simulink model "LQR_MPC_comparison"  (R2023a)
settings: Solver=VariableStepAuto  StartTime=0.0  StopTime=3  RelTol=1e-3
values from neighbouring files (symbols this model uses):
  B_tilda = [sysdis.B(1) Bw_bar(1,1) Bw_bar(1,2); sysdis.B(2) Bw_bar(2,1) Bw_bar(2,2)]    [motor.m]
  D_tilda = [0 0 0 ; 0 0 0]    [motor.m]
  N = 10    [motor.m]    (also in motor_mpc.m = 3; mpc_unconstrained.m)
  Q_LQ = eye(2)    [motor.m]
  R_LQ = 1    [motor.m]
  sysdis = c2d(sys,Ts)    [motor.m]
  Ts = 0.001    [parameters.m]
  u_max = 12    [constraints.m]
  u_min = 0    [constraints.m]
  uBar = -(A(1,1)*(-A(2,2)*nref/A(2,1)) + A(1,2)*nref)*L    [motor.m]
  w = [1 1]'    [parameters.m]
  x0 = [0.2 70.3]'    [motor.m]
  yref = [iref nref]'    [motor.m]
undefined symbols (not defined in the file or in its folder): Kd, motor_mpc, Sd
settings Model: Creator=Diego  LastModifiedBy=paul

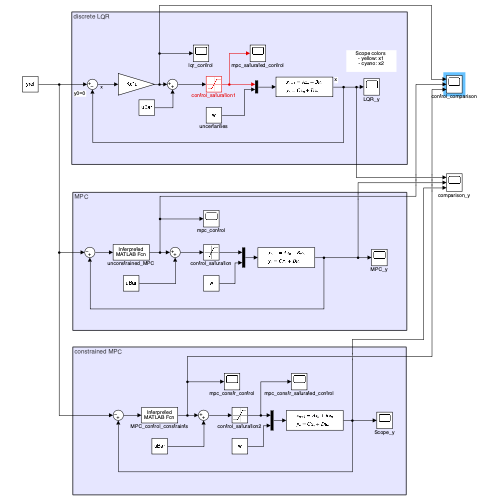
[thumbnail: Simulink's stored preview of the top-level diagram]
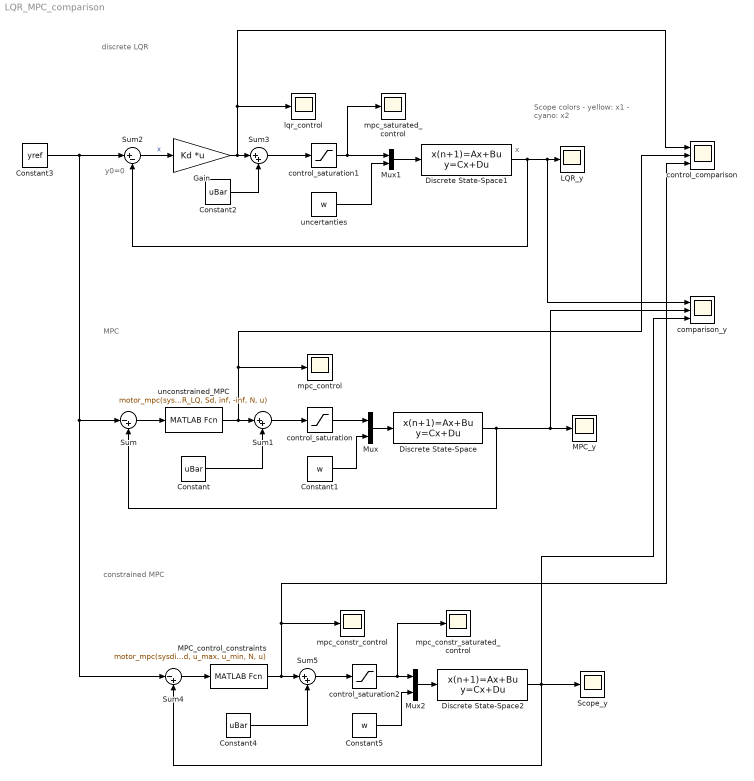
== system LQR_MPC_comparison ==
  note: constrained MPC
  note: discrete LQR
  note: MPC
  note: y0=0
  note: x
  note: Scope colors
      | - yellow: x1
      | - cyano: x2
  Constant : Constant  Value=uBar
  Constant1 : Constant  Value=w
  Constant2 : Constant  Value=uBar
  Constant3 : Constant  Value=yref
  Constant4 : Constant  Value=uBar
  Constant5 : Constant  Value=w
  Discrete State-Space : DiscreteStateSpace  A=sysdis.A  B=B_tilda  C=sysdis.C  D=D_tilda  InitialCondition=x0  SampleTime=Ts
  Discrete State-Space1 : DiscreteStateSpace  A=sysdis.A  B=B_tilda  C=sysdis.C  D=D_tilda  InitialCondition=x0  SampleTime=Ts
  Discrete State-Space2 : DiscreteStateSpace  A=sysdis.A  B=B_tilda  C=sysdis.C  D=D_tilda  InitialCondition=x0  SampleTime=Ts
  Gain : Gain  Gain=Kd  Multiplication=Matrix(K*u)
  LQR_y : Scope
  MPC_control_constraints : MATLABFcn  MATLABFcn=motor_mpc(sysdis.A, sysdis.B, Q_LQ, R_LQ, Sd, u_max, u_min, N, u)  OutputDimensions=1
  MPC_y : Scope
  Mux : Mux  Inputs=2
  Mux1 : Mux  Inputs=2
  Mux2 : Mux  Inputs=2
  Scope_y : Scope
  Sum : Sum  Inputs=|-+
  Sum1 : Sum  Inputs=|++
  Sum2 : Sum  Inputs=|+-
  Sum3 : Sum  Inputs=|++
  Sum4 : Sum  Inputs=|-+
  Sum5 : Sum  Inputs=|++
  comparison_y : Scope  NumInputPorts=3
  control_comparison : Scope  NumInputPorts=3
  control_saturation : Saturate  UpperLimit=u_max  LowerLimit=u_min
  control_saturation1 : Saturate  UpperLimit=u_max  LowerLimit=u_min
  control_saturation2 : Saturate  UpperLimit=u_max  LowerLimit=u_min
  lqr_control : Scope
  mpc_constr_control : Scope
  mpc_constr_saturated_control : Scope
  mpc_control : Scope
  mpc_saturated_control : Scope
  uncertanties : Constant  Value=w
  unconstrained_MPC : MATLABFcn  MATLABFcn=motor_mpc(sysdis.A, sysdis.B, Q_LQ, R_LQ, Sd, inf, -inf, N, u)  OutputDimensions=1
  wires:
  Constant1/1 -> Mux/2
  unconstrained_MPC/1 -> control_comparison/2, mpc_control/1, Sum1/1
  Discrete State-Space/1 -> comparison_y/2, MPC_y/1, Sum/2
  control_saturation/1 -> Mux/1
  Constant/1 -> Sum1/2
  Sum1/1 -> control_saturation/1
  Sum/1 -> unconstrained_MPC/1
  Mux/1 -> Discrete State-Space/1
  Mux1/1 -> Discrete State-Space1/1
  Constant2/1 -> Sum3/2
  Gain/1 -> control_comparison/1, lqr_control/1, Sum3/1
  Sum3/1 -> control_saturation1/1
  Discrete State-Space1/1 -> comparison_y/1, LQR_y/1, Sum2/2
  Sum2/1 -> Gain/1  "x"
  control_saturation1/1 -> Mux1/1, mpc_saturated_control/1
  uncertanties/1 -> Mux1/2
  control_saturation2/1 -> mpc_constr_saturated_control/1, Mux2/1
  Sum4/1 -> MPC_control_constraints/1
  Sum5/1 -> control_saturation2/1
  Constant4/1 -> Sum5/2
  Constant3/1 -> Sum4/1, Sum/1, Sum2/1
  Constant5/1 -> Mux2/2
  Mux2/1 -> Discrete State-Space2/1
  Discrete State-Space2/1 -> comparison_y/3, Scope_y/1, Sum4/2
  MPC_control_constraints/1 -> control_comparison/3, mpc_constr_control/1, Sum5/1
